simulink model "encaout_eml"  (R2014a)
settings: Solver=FixedStepDiscrete  SolverMode=SingleTasking  StartTime=0.0  StopTime=10.0  RelTol=1e-3
settings Model: ExtModeTrigDuration=2  Creator=gcampa  LastModifiedBy=gcampa
settings OptimizationCC: OptimizeModelRefInitCode=on  LifeSpan=1
settings DebuggingCC: UnderspecifiedInitializationDetection=Classic  SolverPrmCheckMsg=none  FrameProcessingCompatibilityMsg=error  StateNameClashWarn=warning
settings HardwareCC: ProdBitPerInt=16  ProdBitPerPointer=8  ProdIntDivRoundTo=Zero  ProdEndianess=LittleEndian  ProdWordSize=8  ProdHWDeviceType=Atmel->AVR
settings RTWCC: SystemTargetFile=realtime.tlc  GenerateMakefile=off  TemplateMakefile=realtime.tmf  Description=Run on Target Hardware  RTWVerbose=off  ProcessScript=realtime_make_rtw_hook  CustomSource=..\src\encoder_arduino.cpp ..\src\aout_arduino.cpp
settings STFCustomTargetCC: TargetLibSuffix=.a  GenerateSampleERTMain=on  ConcurrentExecutionCompliant=off  GeneratePreprocessorConditionals=Use local settings  ERTCustomFileBanners=on  SupportNonInlinedSFcns=off  SupportVariableSizeSignals=on  MATLABClassNameForMDSCustomization=Simulink.SoftwareTarget.ERTCustomization  GRTInterface=off  SystemTargetFile=realtime.tlc
settings ERTTargetCC: CombineOutputUpdateFcns=off  SupportContinuousTime=on  SupportVariableSizeSignals=on  ExtModeTransport=3  ExtModeMexFile=ext_serial_win32_comm  ExtModeMexArgs=0 1 9600  ERTSrcFileBannerTemplate=realtime_code_template.cgt  ERTHdrFileBannerTemplate=realtime_code_template.cgt  ERTDataSrcFileTemplate=realtime_code_template.cgt  ERTDataHdrFileTemplate=realtime_code_template.cgt  ERTCustomFileTemplate=realtime_file_process.tlc

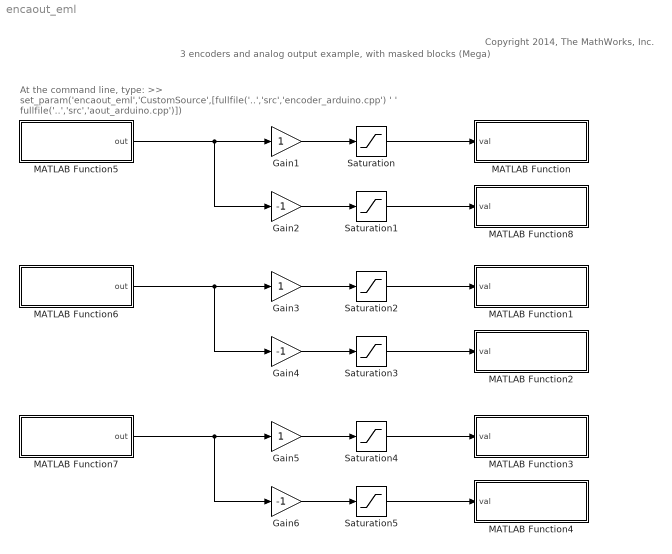
== system encaout_eml ==
  note: 3 encoders and analog output example, with masked blocks (Mega)
  note: At the command line, type:
      | >> set_param('encaout_eml','CustomSource',[fullfile('..','src','encoder_arduino.cpp') ' ' fullfile('..','src','aout_arduino.cpp')])
  note: Copyright 2014, The MathWorks, Inc.
  Gain1 : Gain  OutDataTypeStr=Inherit: Same as input
  Gain2 : Gain  Gain=-1  OutDataTypeStr=Inherit: Same as input
  Gain3 : Gain  OutDataTypeStr=Inherit: Same as input
  Gain4 : Gain  Gain=-1  OutDataTypeStr=Inherit: Same as input
  Gain5 : Gain  OutDataTypeStr=Inherit: Same as input
  Gain6 : Gain  Gain=-1  OutDataTypeStr=Inherit: Same as input
  MATLAB Function : MATLAB Function  TreatAsAtomicUnit=on  mask(Analog Write){pin=9, T=0.05}
      mask prompts: T "Sample Time"
      mask help:
      | Every time this block is executed it gets an analog value from 0 or 255 at its input and writes it (via PWM) to a given pin. Basically a square 490Hz waveform is generated with a duty cycle from 0 (corresponding to 0 V) to 255 (corresponding to 5V).
      |
      | The first parameter in the is the number of the pin where the analog output needs to be performed. The second parameter is the sample time.
      |
      | Note that if this block gets copied to a new model, then the file "aout_arduino.cpp" must be added to the CustomSource field of the new model using the "set_param" instruction. See the guide for more info.
  MATLAB Function1 : MATLAB Function  TreatAsAtomicUnit=on  mask(Analog Write){pin=11, T=0.05}
      mask prompts: T "Sample Time"
      mask help:
      | Every time this block is executed it gets an analog value from 0 or 255 at its input and writes it (via PWM) to a given pin. Basically a square 490Hz waveform is generated with a duty cycle from 0 (corresponding to 0 V) to 255 (corresponding to 5V).
      |
      | The first parameter in the is the number of the pin where the analog output needs to be performed. The second parameter is the sample time.
      |
      | Note that if this block gets copied to a new model, then the file "aout_arduino.cpp" must be added to the CustomSource field of the new model using the "set_param" instruction. See the guide for more info.
  MATLAB Function2 : MATLAB Function  TreatAsAtomicUnit=on  mask(Analog Write){pin=12, T=0.05}
      mask prompts: T "Sample Time"
      mask help:
      | Every time this block is executed it gets an analog value from 0 or 255 at its input and writes it (via PWM) to a given pin. Basically a square 490Hz waveform is generated with a duty cycle from 0 (corresponding to 0 V) to 255 (corresponding to 5V).
      |
      | The first parameter in the is the number of the pin where the analog output needs to be performed. The second parameter is the sample time.
      |
      | Note that if this block gets copied to a new model, then the file "aout_arduino.cpp" must be added to the CustomSource field of the new model using the "set_param" instruction. See the guide for more info.
  MATLAB Function3 : MATLAB Function  TreatAsAtomicUnit=on  mask(Analog Write){pin=5, T=0.05}
      mask prompts: T "Sample Time"
      mask help:
      | Every time this block is executed it gets an analog value from 0 or 255 at its input and writes it (via PWM) to a given pin. Basically a square 490Hz waveform is generated with a duty cycle from 0 (corresponding to 0 V) to 255 (corresponding to 5V).
      |
      | The first parameter in the is the number of the pin where the analog output needs to be performed. The second parameter is the sample time.
      |
      | Note that if this block gets copied to a new model, then the file "aout_arduino.cpp" must be added to the CustomSource field of the new model using the "set_param" instruction. See the guide for more info.
  MATLAB Function4 : MATLAB Function  TreatAsAtomicUnit=on  mask(Analog Write){pin=6, T=0.05}
      mask prompts: T "Sample Time"
      mask help:
      | Every time this block is executed it gets an analog value from 0 or 255 at its input and writes it (via PWM) to a given pin. Basically a square 490Hz waveform is generated with a duty cycle from 0 (corresponding to 0 V) to 255 (corresponding to 5V).
      |
      | The first parameter in the is the number of the pin where the analog output needs to be performed. The second parameter is the sample time.
      |
      | Note that if this block gets copied to a new model, then the file "aout_arduino.cpp" must be added to the CustomSource field of the new model using the "set_param" instruction. See the guide for more info.
  MATLAB Function5 : MATLAB Function  TreatAsAtomicUnit=on  mask(Encoder Read){enc=0, pinA=2, pinB=3, T=0.05}
      mask prompts: enc "Encoder Number (0, 1 or 2)"; pinA "Pin A"; pinB "Pin B"; T "Sample TIme"
      mask help:
      | At initialization time, this block attaches interrupt service routines (written in eml_enc_src.c) to the two pins (pinA and pinB) to which the encoder is connected (the "common" central pin a.k.a. pinC of the encoder should be connected to ground). After that, when the encoder rotates the interrupts service routines update the encoder position. The encoder position is then set as output of the block every time the block is executed.
      |
      | The first parameter is the encoder identifier, must be either 0, 1 or 2. PinA and PinB are the pins to which the encoder is attached. The allowed pins are 2 and 3 on the Uno board and 2,3,18,19,20,21 on the Mega board. The last parameter is the Sample Time.
      |
      | Note that if this block gets copied to a new model, then the file "encoder_arduino.cpp" must be added to the CustomSource field of the new model using the "set_param" instruction. See the guide for more info.
  MATLAB Function6 : MATLAB Function  TreatAsAtomicUnit=on  mask(Encoder Read){enc=1, pinA=18, pinB=19, T=0.05}
      mask prompts: enc "Encoder Number (0, 1 or 2)"; pinA "Pin A"; pinB "Pin B"; T "Sample TIme"
      mask help:
      | At initialization time, this block attaches interrupt service routines (written in eml_enc_src.c) to the two pins (pinA and pinB) to which the encoder is connected (the "common" central pin a.k.a. pinC of the encoder should be connected to ground). After that, when the encoder rotates the interrupts service routines update the encoder position. The encoder position is then set as output of the block every time the block is executed.
      |
      | The first parameter is the encoder identifier, must be either 0, 1 or 2. PinA and PinB are the pins to which the encoder is attached. The allowed pins are 2 and 3 on the Uno board and 2,3,18,19,20,21 on the Mega board. The last parameter is the Sample Time.
      |
      | Note that if this block gets copied to a new model, then the file "encoder_arduino.cpp" must be added to the CustomSource field of the new model using the "set_param" instruction. See the guide for more info.
  MATLAB Function7 : MATLAB Function  TreatAsAtomicUnit=on  mask(Encoder Read){enc=2, pinA=20, pinB=21, T=0.05}
      mask prompts: enc "Encoder Number (0, 1 or 2)"; pinA "Pin A"; pinB "Pin B"; T "Sample TIme"
      mask help:
      | At initialization time, this block attaches interrupt service routines (written in eml_enc_src.c) to the two pins (pinA and pinB) to which the encoder is connected (the "common" central pin a.k.a. pinC of the encoder should be connected to ground). After that, when the encoder rotates the interrupts service routines update the encoder position. The encoder position is then set as output of the block every time the block is executed.
      |
      | The first parameter is the encoder identifier, must be either 0, 1 or 2. PinA and PinB are the pins to which the encoder is attached. The allowed pins are 2 and 3 on the Uno board and 2,3,18,19,20,21 on the Mega board. The last parameter is the Sample Time.
      |
      | Note that if this block gets copied to a new model, then the file "encoder_arduino.cpp" must be added to the CustomSource field of the new model using the "set_param" instruction. See the guide for more info.
  MATLAB Function8 : MATLAB Function  TreatAsAtomicUnit=on  mask(Analog Write){pin=10, T=0.05}
      mask prompts: T "Sample Time"
      mask help:
      | Every time this block is executed it gets an analog value from 0 or 255 at its input and writes it (via PWM) to a given pin. Basically a square 490Hz waveform is generated with a duty cycle from 0 (corresponding to 0 V) to 255 (corresponding to 5V).
      |
      | The first parameter in the is the number of the pin where the analog output needs to be performed. The second parameter is the sample time.
      |
      | Note that if this block gets copied to a new model, then the file "aout_arduino.cpp" must be added to the CustomSource field of the new model using the "set_param" instruction. See the guide for more info.
  Saturation{,1..5} (6 alike) : Saturate  UpperLimit=255  LowerLimit=0  OutDataTypeStr=Inherit: Inherit via back propagation
  wires:
  Saturation/1 -> MATLAB Function/1(val)
  Gain1/1 -> Saturation/1
  MATLAB Function5/1(out) -> Gain2/1, Gain1/1
  Gain2/1 -> Saturation1/1
  Saturation1/1 -> MATLAB Function8/1(val)
  Saturation2/1 -> MATLAB Function1/1(val)
  Gain3/1 -> Saturation2/1
  MATLAB Function6/1(out) -> Gain3/1, Gain4/1
  Gain4/1 -> Saturation3/1
  Saturation3/1 -> MATLAB Function2/1(val)
  Saturation4/1 -> MATLAB Function3/1(val)
  Gain5/1 -> Saturation4/1
  MATLAB Function7/1(out) -> Gain6/1, Gain5/1
  Gain6/1 -> Saturation5/1
  Saturation5/1 -> MATLAB Function4/1(val)

== matlab function encaout_eml/MATLAB Function7 ==
  settings: updateMethod=DISCRETE  sampleTime=T
  data: enc parameter int32; out output; pinA parameter int32; pinB parameter uint8
function out = encoderRead(enc,pinA,pinB)
%#codegen

persistent initflag;
out=0;

if strcmp(coder.target, 'rtw'),
    
    if isempty(initflag),
        % Initialize step
        coder.ceval('enc_init',int16(enc),int16(pinA),int16(pinB));
        initflag = 1;
    else
        % output Step
        out=coder.ceval('enc_output',int16(enc));
    end
    
end

== matlab function encaout_eml/MATLAB Function ==
  settings: updateMethod=DISCRETE  sampleTime=T
  data: pin parameter; val input
function analogWrite(pin,val)
%#codegen

persistent initflag;

if strcmp(coder.target, 'rtw'),
    
    if isempty(initflag),
        % Initialize step
        coder.ceval('aout_init',uint8(pin));
        initflag = 1;
    else
        % output Step
        coder.ceval('aout_output', uint8(pin), uint8(val));
    end
    
end

== matlab function encaout_eml/MATLAB Function1 ==
  settings: updateMethod=DISCRETE  sampleTime=T
  data: pin parameter; val input
function analogWrite(pin,val)
%#codegen

persistent initflag;

if strcmp(coder.target, 'rtw'),
    
    if isempty(initflag),
        % Initialize step
        coder.ceval('aout_init',uint8(pin));
        initflag = 1;
    else
        % output Step
        coder.ceval('aout_output', uint8(pin), uint8(val));
    end
    
end

== matlab function encaout_eml/MATLAB Function2 ==
  settings: updateMethod=DISCRETE  sampleTime=T
  data: pin parameter; val input
function analogWrite(pin,val)
%#codegen

persistent initflag;

if strcmp(coder.target, 'rtw'),
    
    if isempty(initflag),
        % Initialize step
        coder.ceval('aout_init',uint8(pin));
        initflag = 1;
    else
        % output Step
        coder.ceval('aout_output', uint8(pin), uint8(val));
    end
    
end

== matlab function encaout_eml/MATLAB Function3 ==
  settings: updateMethod=DISCRETE  sampleTime=T
  data: pin parameter; val input
function analogWrite(pin,val)
%#codegen

persistent initflag;

if strcmp(coder.target, 'rtw'),
    
    if isempty(initflag),
        % Initialize step
        coder.ceval('aout_init',uint8(pin));
        initflag = 1;
    else
        % output Step
        coder.ceval('aout_output', uint8(pin), uint8(val));
    end
    
end

== matlab function encaout_eml/MATLAB Function6 ==
  settings: updateMethod=DISCRETE  sampleTime=T
  data: enc parameter int32; out output; pinA parameter int32; pinB parameter uint8
function out = encoderRead(enc,pinA,pinB)
%#codegen

persistent initflag;
out=0;

if strcmp(coder.target, 'rtw'),
    
    if isempty(initflag),
        % Initialize step
        coder.ceval('enc_init',int16(enc),int16(pinA),int16(pinB));
        initflag = 1;
    else
        % output Step
        out=coder.ceval('enc_output',int16(enc));
    end
    
end

== matlab function encaout_eml/MATLAB Function4 ==
  settings: updateMethod=DISCRETE  sampleTime=T
  data: pin parameter; val input
function analogWrite(pin,val)
%#codegen

persistent initflag;

if strcmp(coder.target, 'rtw'),
    
    if isempty(initflag),
        % Initialize step
        coder.ceval('aout_init',uint8(pin));
        initflag = 1;
    else
        % output Step
        coder.ceval('aout_output', uint8(pin), uint8(val));
    end
    
end

== matlab function encaout_eml/MATLAB Function5 ==
  settings: updateMethod=DISCRETE  sampleTime=T
  data: enc parameter int32; out output; pinA parameter int32; pinB parameter uint8
function out = encoderRead(enc,pinA,pinB)
%#codegen

persistent initflag;
out=0;

if strcmp(coder.target, 'rtw'),
    
    if isempty(initflag),
        % Initialize step
        coder.ceval('enc_init',int16(enc),int16(pinA),int16(pinB));
        initflag = 1;
    else
        % output Step
        out=coder.ceval('enc_output',int16(enc));
    end
    
end

== matlab function encaout_eml/MATLAB Function8 ==
  settings: updateMethod=DISCRETE  sampleTime=T
  data: pin parameter; val input
function analogWrite(pin,val)
%#codegen

persistent initflag;

if strcmp(coder.target, 'rtw'),
    
    if isempty(initflag),
        % Initialize step
        coder.ceval('aout_init',uint8(pin));
        initflag = 1;
    else
        % output Step
        coder.ceval('aout_output', uint8(pin), uint8(val));
    end
    
end
